simulink model "prob7_subsystem"  (R2020b)
settings: Solver=VariableStepAuto  StartTime=0.0  StopTime=10.0  RelTol=1e-3
settings Model: Creator=Gopinath Murugan  LastModifiedBy=Gopinath Murugan

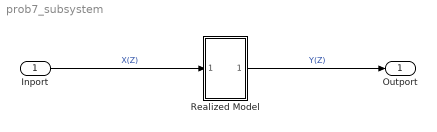
== system prob7_subsystem ==
  Inport : Inport
  Realized Model : Subsystem
  Outport : Outport
  wires:
  Inport/1 -> Realized Model/1(In1)  "X(Z)"
  Realized Model/1(Out1) -> Outport/1  "Y(Z)"

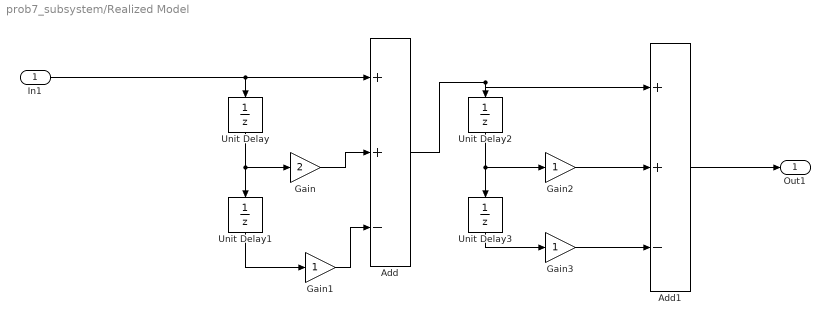
== system prob7_subsystem/Realized Model ==
  In1 : Inport
  Add : Sum  Inputs=++-
  Add1 : Sum  Inputs=++-
  Gain : Gain  Gain=2
  Gain1 : Gain
  Gain2 : Gain
  Gain3 : Gain
  Unit Delay{,1..3} (4 alike) : UnitDelay  SampleTime=-1  HasFrameUpgradeWarning=on
  Out1 : Outport
  wires:
  Gain2/1 -> Add1/2
  Unit Delay/1 -> Gain/1, Unit Delay1/1
  In1/1 -> Unit Delay/1, Add/1
  Unit Delay2/1 -> Gain2/1, Unit Delay3/1
  Unit Delay1/1 -> Gain1/1
  Gain/1 -> Add/2
  Unit Delay3/1 -> Gain3/1
  Add/1 -> Add1/1, Unit Delay2/1
  Gain3/1 -> Add1/3
  Gain1/1 -> Add/3
  Add1/1 -> Out1/1
